simulink model "testSampleModelRef"  (R2023b)
settings: Solver=VariableStepAuto  StartTime=0.0  StopTime=10.0  RelTol=1e-3
settings Model: Creator=peterc  LastModifiedBy=peterc

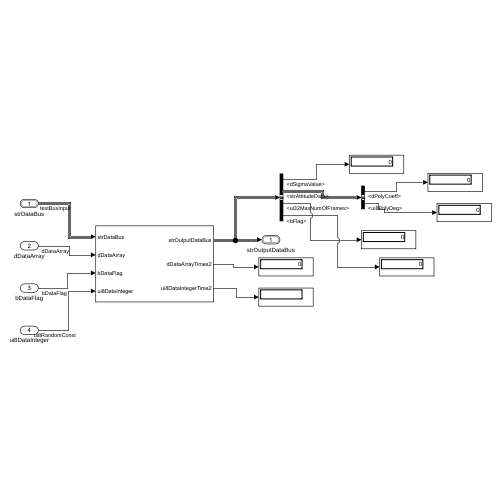
[thumbnail: Simulink's stored preview of the top-level diagram]
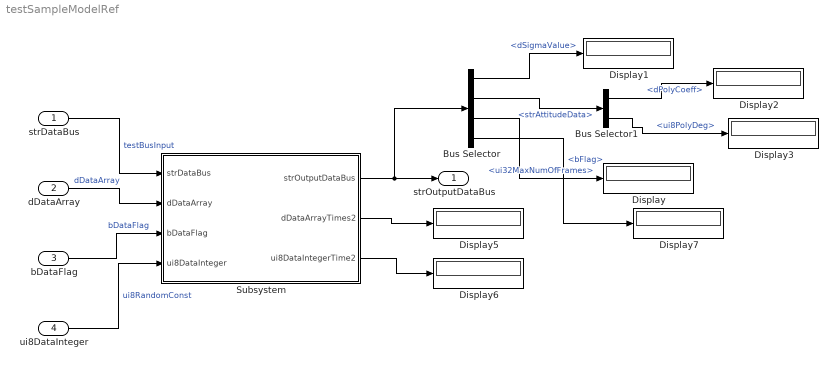
== system testSampleModelRef ==
  strDataBus : Inport  OutDataTypeStr=Bus: bus_testBusWithExample
  dDataArray : Inport  Port=2  OutDataTypeStr=double  PortDimensions=[9,9]
  bDataFlag : Inport  Port=3  OutDataTypeStr=boolean
  ui8DataInteger : Inport  Port=4  OutDataTypeStr=uint8
  Bus Selector : BusSelector  OutputSignals=dSigmaValue,strAttitudeData,ui32MaxNumOfFrames,bFlag
  Bus Selector1 : BusSelector  OutputSignals=dPolyCoeff,ui8PolyDeg
  Display{,1..3,5..7} (7 alike) : Display
  Subsystem : Subsystem
  strOutputDataBus : Outport  OutDataTypeStr=Bus: bus_testBusWithExample
  wires:
  strDataBus/1 -> Subsystem/1(strDataBus)  "testBusInput"
  dDataArray/1 -> Subsystem/2(dDataArray)  "dDataArray"
  bDataFlag/1 -> Subsystem/3(bDataFlag)  "bDataFlag"
  ui8DataInteger/1 -> Subsystem/4(ui8DataInteger)  "ui8RandomConst"
  Subsystem/1(strOutputDataBus) -> Bus Selector/1, strOutputDataBus/1
  Bus Selector/1 -> Display1/1  "<dSigmaValue>"
  Bus Selector/2 -> Bus Selector1/1  "<strAttitudeData>"
  Bus Selector/3 -> Display/1  "<ui32MaxNumOfFrames>"
  Bus Selector1/1 -> Display2/1  "<dPolyCoeff>"
  Bus Selector1/2 -> Display3/1  "<ui8PolyDeg>"
  Subsystem/2(dDataArrayTimes2) -> Display5/1
  Subsystem/3(ui8DataIntegerTime2) -> Display6/1
  Bus Selector/4 -> Display7/1  "<bFlag>"

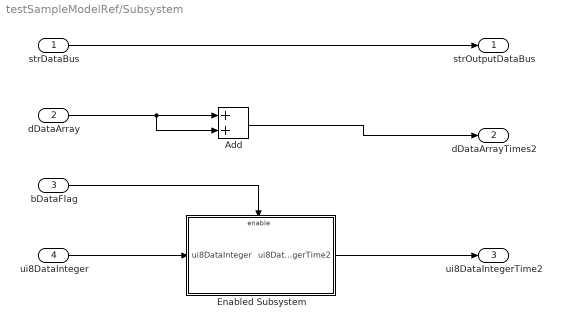
== system testSampleModelRef/Subsystem ==
  strDataBus : Inport  OutDataTypeStr=Bus: bus_testBusWithExample
  dDataArray : Inport  Port=2
  bDataFlag : Inport  Port=3
  ui8DataInteger : Inport  Port=4
  Add : Sum
  Enabled Subsystem : Subsystem  TreatAsAtomicUnit=on
  strOutputDataBus : Outport  OutDataTypeStr=Bus: bus_testBusWithExample
  dDataArrayTimes2 : Outport  Port=2
  ui8DataIntegerTime2 : Outport  Port=3
  wires:
  dDataArray/1 -> Add/2, Add/1
  strDataBus/1 -> strOutputDataBus/1
  bDataFlag/1 -> Enabled Subsystem/Enable
  ui8DataInteger/1 -> Enabled Subsystem/1(ui8DataInteger)
  Add/1 -> dDataArrayTimes2/1
  Enabled Subsystem/1(ui8DataIntegerTime2) -> ui8DataIntegerTime2/1

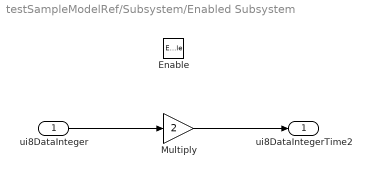
== system testSampleModelRef/Subsystem/Enabled Subsystem ==
  ui8DataInteger : Inport
  Enable : EnablePort
  Multiply : Gain  Gain=2  ParamDataTypeStr=Inherit: Same as input
  ui8DataIntegerTime2 : Outport
  wires:
  ui8DataInteger/1 -> Multiply/1
  Multiply/1 -> ui8DataIntegerTime2/1
